simulink model "example_9"  (R2022b)
settings: Solver=VariableStepAuto  StartTime=0.0  StopTime=10.0  RelTol=1e-3
settings Model: Creator=Mahadevu Sudheer  LastModifiedBy=Mahadevu Sudheer

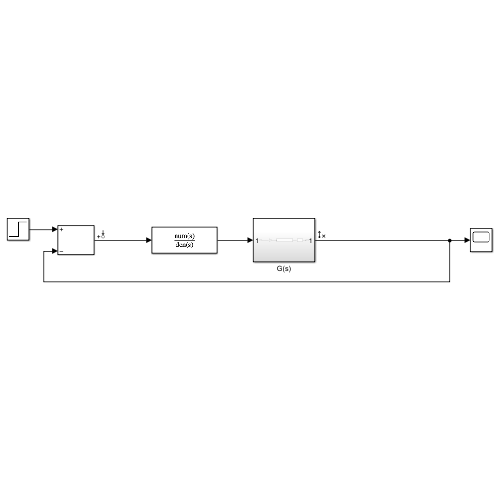
[thumbnail: Simulink's stored preview of the top-level diagram]
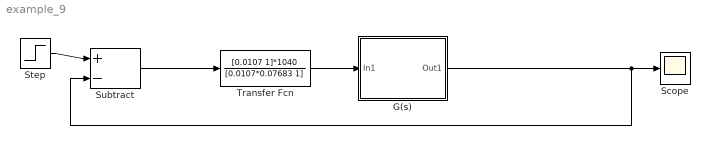
== system example_9 ==
  G(s) : Subsystem
  Scope : Scope
  Step : Step  Time=0  SampleTime=0
  Subtract : Sum  Inputs=+||-
  Transfer Fcn : TransferFcn  Numerator=[0.0107 1]*1040  Denominator=[0.0107*0.07683 1]
  wires:
  Step/1 -> Subtract/1
  G(s)/1(Out1) -> Subtract/2, Scope/1
  Transfer Fcn/1 -> G(s)/1(In1)
  Subtract/1 -> Transfer Fcn/1

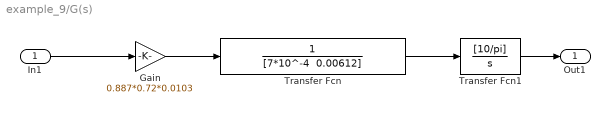
== system example_9/G(s) ==
  In1 : Inport
  Gain : Gain  Gain=0.887*0.72*0.0103
  Transfer Fcn : TransferFcn  Denominator="[7*10^-4  0.00612]"
  Transfer Fcn1 : TransferFcn  Numerator=[10/pi]  Denominator=[1 0]
  Out1 : Outport
  wires:
  In1/1 -> Gain/1
  Transfer Fcn/1 -> Transfer Fcn1/1
  Gain/1 -> Transfer Fcn/1
  Transfer Fcn1/1 -> Out1/1
